simulink model "Case1simulimk"  (R2022b)
settings: Solver=FixedStepAuto  StartTime=0.0  StopTime=8  FixedStep=1e-4  RelTol=1e-3  EnableMultiTasking=on
undefined symbols (not defined in the file): Fcc, Kb, P, rho, T, x0
settings Model: Creator=sf  LastModifiedBy=sf
settings ModelReferenceCC: EnableRefExpFcnMdlSchedulingChecks=on

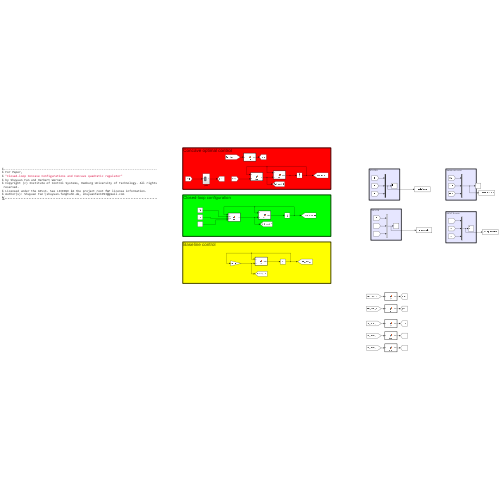
[thumbnail: Simulink's stored preview of the top-level diagram]
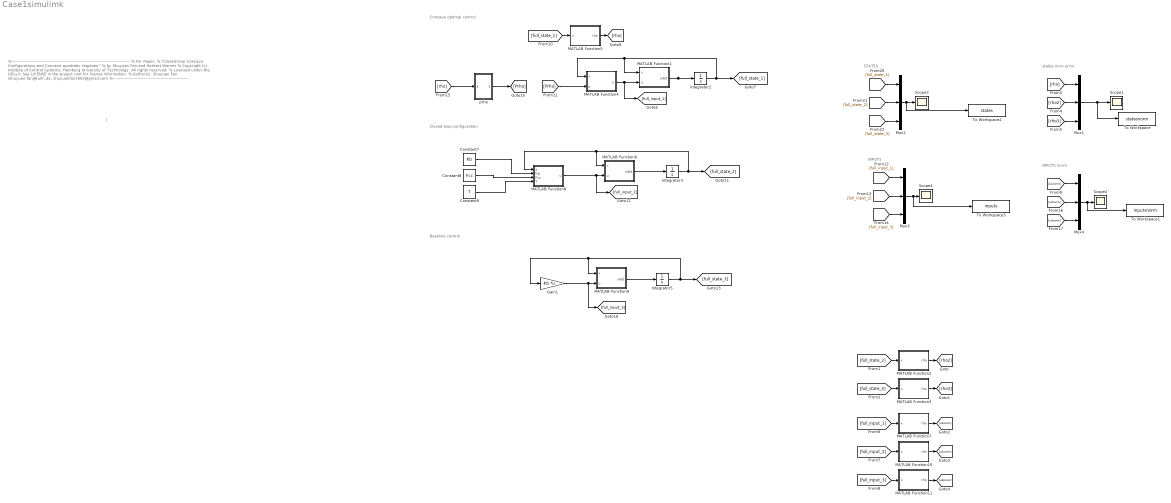
== system Case1simulimk ==
  note: )
  note: %-----------------------------------------------------------------------------------------
      | % For Paper,
      | % "Closed-loop Concave Configurations and Concave quadratic regulator"
      | % by Shuyuan Fan and Herbert Werner
      | % Copyright (c) Institute of Control Systems, Hamburg University of Technology. All rights reserved.
      | % Licensed under the GPLv3. See LICENSE in the project root for license information.
      | % Author(s): Shuyuan Fan (shuyuan.fan@tuhh.de, shuyuanfan1993@gmail.com
      | %---------------------------------------------------------
  note: INPUTS
  note: STATES
  note: Baseline control
  note: Concave optimal control
  note: Closed-loop configuration
  note: states norn error
  note: INPUTS norm
  Constant7 : Constant  Value=Kb
  Constant8 : Constant  Value=Fcc
  Constant9 : Constant  Value=T
  Gain1 : Gain  Gain=-Kb  Multiplication=Matrix(K*u)
  Integrator2 : Integrator  InitialCondition=x0
  Integrator3 : Integrator  InitialCondition=x0
  Integrator5 : Integrator  InitialCondition=x0
  MATLAB Function1 : MATLAB Function  TreatAsAtomicUnit=on
  MATLAB Function10 : MATLAB Function  TreatAsAtomicUnit=on
  MATLAB Function11 : MATLAB Function  TreatAsAtomicUnit=on
  MATLAB Function2 : MATLAB Function  TreatAsAtomicUnit=on
  MATLAB Function3 : MATLAB Function  TreatAsAtomicUnit=on
  MATLAB Function4 : MATLAB Function  TreatAsAtomicUnit=on
  MATLAB Function5 : MATLAB Function  TreatAsAtomicUnit=on
  MATLAB Function6 : MATLAB Function  TreatAsAtomicUnit=on
  MATLAB Function7 : MATLAB Function  TreatAsAtomicUnit=on
  MATLAB Function8 : MATLAB Function  TreatAsAtomicUnit=on
  MATLAB Function9 : MATLAB Function  TreatAsAtomicUnit=on
  Mux{1..4} (4 alike) : Mux  Inputs=3
  Scope{1..4} (4 alike) : Scope
  To Workspace : ToWorkspace  VariableName=statesnorm  SaveFormat=Timeseries  SampleTime=-1
  To Workspace1 : ToWorkspace  VariableName=inputsnorm  SaveFormat=Timeseries  SampleTime=-1
  To Workspace2 : ToWorkspace  VariableName=states  SaveFormat=Timeseries  SampleTime=-1
  To Workspace3 : ToWorkspace  VariableName=inputs  SaveFormat=Timeseries  SampleTime=-1
  prho : Subsystem
  wires:
  Mux3/1 -> To Workspace3/1, Scope4/1
  MATLAB Function5/1(rho) -> [rho]
  [full_state_1] -> Mux2/1
  Integrator5/1 -> MATLAB Function9/1(x), Gain1/1, [full_state_3]
  MATLAB Function6/1(xdot) -> Integrator3/1
  [full_state_2] -> Mux2/2
  Integrator2/1 -> MATLAB Function1/1(x), MATLAB Function4/1(x), [full_state_1]
  MATLAB Function9/1(xdot) -> Integrator5/1
  [full_state_3] -> Mux2/3
  Integrator3/1 -> MATLAB Function6/1(x), MATLAB Function8/1(x), [full_state_2]
  Gain1/1 -> MATLAB Function9/2(u), [full_input_3]
  Mux2/1 -> To Workspace2/1, Scope3/1
  [rho] -> prho/1(In1)
  prho/1(Out1) -> [Prho]
  [full_input_1] -> Mux3/1
  MATLAB Function8/1(u) -> MATLAB Function6/2(u), [full_input_2]
  [full_input_3] -> Mux3/3
  [full_state_1] -> MATLAB Function5/1(x)
  MATLAB Function4/1(u) -> MATLAB Function1/2(u), [full_input_1]
  MATLAB Function1/1(xdot) -> Integrator2/1
  [Prho] -> MATLAB Function4/2(p)
  [full_input_2] -> Mux3/2
  Constant7/1 -> MATLAB Function8/2(Kb)
  Constant8/1 -> MATLAB Function8/3(Fcc)
  Constant9/1 -> MATLAB Function8/4(T)
  [full_state_2] -> MATLAB Function2/1(x)
  [full_state_3] -> MATLAB Function3/1(x)
  MATLAB Function2/1(rho) -> [rho2]
  MATLAB Function3/1(rho) -> [rho3]
  [rho2] -> Mux1/2
  Mux1/1 -> To Workspace/1, Scope1/1
  [rho3] -> Mux1/3
  [rho] -> Mux1/1
  MATLAB Function7/1(rho) -> [u1norm]
  [full_input_2] -> MATLAB Function10/1(x)
  [full_input_1] -> MATLAB Function7/1(x)
  MATLAB Function10/1(rho) -> [u2norm]
  [full_input_3] -> MATLAB Function11/1(x)
  MATLAB Function11/1(rho) -> [u3norm]
  [u1norm] -> Mux4/1
  [u2norm] -> Mux4/2
  [u3norm] -> Mux4/3
  Mux4/1 -> To Workspace1/1, Scope2/1

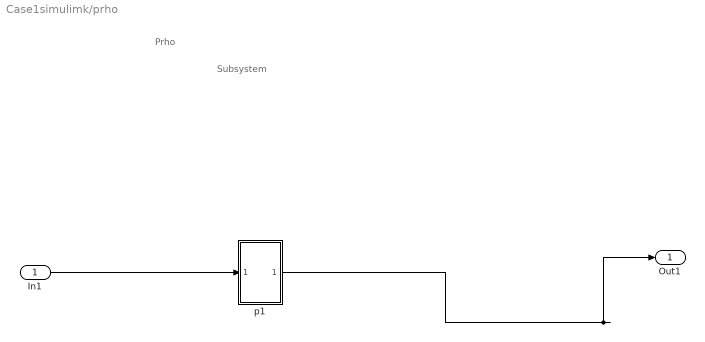
== system Case1simulimk/prho ==
  note: Prho
  note: Subsystem
  In1 : Inport
  p1 : Subsystem
  Out1 : Outport
  wires:
  In1/1 -> p1/1(In1)
  p1/1(Out1) -> Out1/1

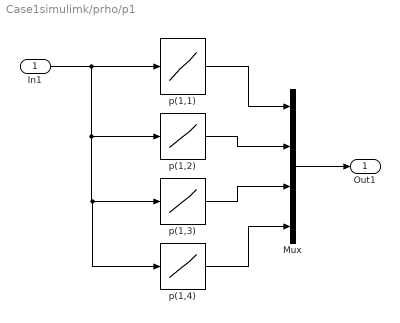
== system Case1simulimk/prho/p1 ==
  In1 : Inport
  Mux : Mux
  p(1,1) : Lookup_n-D  NumberOfTableDimensions=1  BreakpointsForDimension1=rho  Table=P(:,1)  InterpMethod=Linear Lagrange  InternalRulePriority=Speed  RndMeth=Simplest
  p(1,2) : Lookup_n-D  NumberOfTableDimensions=1  BreakpointsForDimension1=rho  Table=P(:,2)  InterpMethod=Linear Lagrange  InternalRulePriority=Speed  RndMeth=Simplest
  p(1,3) : Lookup_n-D  NumberOfTableDimensions=1  BreakpointsForDimension1=rho  Table=P(:,2)  InterpMethod=Linear Lagrange  InternalRulePriority=Speed  RndMeth=Simplest
  p(1,4) : Lookup_n-D  NumberOfTableDimensions=1  BreakpointsForDimension1=rho  Table=P(:,4)  InterpMethod=Linear Lagrange  InternalRulePriority=Speed  RndMeth=Simplest
  Out1 : Outport
  wires:
  p(1,2)/1 -> Mux/2
  p(1,4)/1 -> Mux/4
  In1/1 -> p(1,4)/1, p(1,3)/1, p(1,2)/1, p(1,1)/1
  p(1,1)/1 -> Mux/1
  p(1,3)/1 -> Mux/3
  Mux/1 -> Out1/1

== matlab function Case1simulimk/MATLAB Function1 ==
  data: x input; xdot output; u input
function xdot = fcn(x,u)
A = [-1 1;-1 1];
B =  [1, 1; 2, 1];

xdot = A*x+B*u;

end

== matlab function Case1simulimk/MATLAB Function2 ==
  data: x input; rho output
function rho = fcn(x)

rho = sqrt(x'*x);

== matlab function Case1simulimk/MATLAB Function3 ==
  data: x input; rho output
function rho = fcn(x)

rho = sqrt(x'*x);

== matlab function Case1simulimk/MATLAB Function10 ==
  data: x input; rho output
function rho = fcn(x)

rho = sqrt(x'*x);

== matlab function Case1simulimk/MATLAB Function7 ==
  data: x input; rho output
function rho = fcn(x)

rho = sqrt(x'*x);

== matlab function Case1simulimk/MATLAB Function4 ==
  data: x input; u output; p input
function u= fcn(x,p)
R = diag([1,1]);
% system matrix
A = [-1 1;-1 1];
B = [1, 1; 2,1];

p_ = reshape(p,[2,2]);
P = p_';
R_inv = inv(R);
u = -R_inv*B'*P*x;

== matlab function Case1simulimk/MATLAB Function6 ==
  data: x input; xdot output; u input
function xdot = fcn(x,u)
A = [-1 1;-1 1];
B =  [1, 1; 2, 1];

xdot = A*x+B*u;

end

== matlab function Case1simulimk/MATLAB Function11 ==
  data: x input; rho output
function rho = fcn(x)

rho = sqrt(x'*x);

== matlab function Case1simulimk/MATLAB Function5 ==
  data: x input; rho output
function rho = fcn(x)

rho = sqrt(x'*x);

== matlab function Case1simulimk/MATLAB Function9 ==
  data: x input; xdot output; u input
function xdot = fcn(x,u)
A = [-1 1;-1 1];
B =  [1, 1; 2, 1];

xdot = A*x+B*u;

end

== matlab function Case1simulimk/MATLAB Function8 ==
  data: x input; u output; Kb input; Fcc input; T input
function u= fcn(x,Kb,Fcc,T)

% system matrix
A = [-1 1;-1 1];
B = [1, 1; 2,1];

% baseline controller
%Kb = reshape(Kb,[2,2]);
Aclb = A-B*Kb;

% transformation matrix

%T = reshape(T,[2,2]);

% xtilde

xtilde = T*x;

%rho

rho1  = abs(xtilde(1));

rho2 = abs(xtilde(2));

%concave factor
% parameters of concave factor
k1min = Fcc(1); k1max = Fcc(2); beta1 = Fcc(3); eta1 = Fcc(4);
k2min = Fcc(5); k2max = Fcc(6); beta2 = Fcc(7); eta2 = Fcc(8);

fc1 = fcs(rho1,k1min,k1max,beta1,eta1);
fc2 = fcs(rho2,k2min,k2max,beta2,eta2);

Fc = diag([fc1,fc2]);

%Controlgain
Bstar = B'*B;
Kn = inv(Bstar)*B'*(A-Aclb*inv(T)*Fc*T);

% calculate input
u  = -Kn*x;
end
